simulink model "myModel"  (R2025a)
settings: Solver=VariableStepAuto  StartTime=0.0  StopTime=10.0  RelTol=1e-3

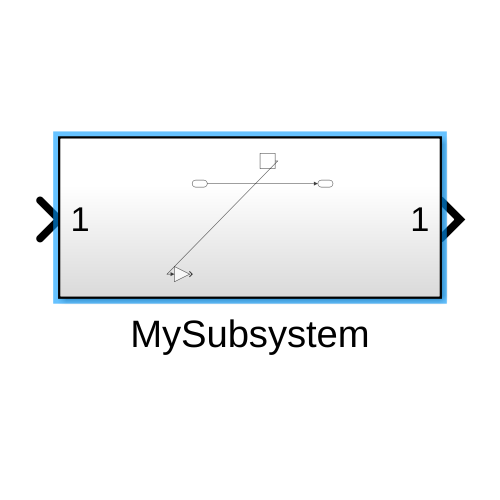
[thumbnail: Simulink's stored preview of the top-level diagram]
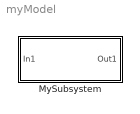
== system myModel ==
  MySubsystem : Subsystem

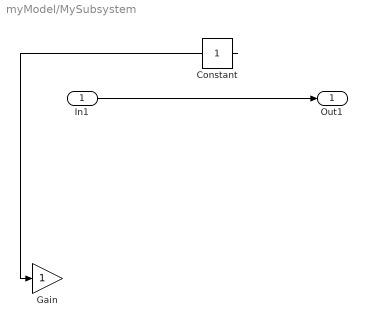
== system myModel/MySubsystem ==
  In1 : Inport
  Constant : Constant
  Gain : Gain
  Out1 : Outport
  wires:
  In1/1 -> Out1/1
  Constant/1 -> Gain/1
